simulink model "soal1ghesmatb"  (R2019b)
settings: Solver=VariableStepAuto  StartTime=0.0  StopTime=10.0  RelTol=1e-3
libraries: simulink x2
settings Model: Creator=user  LastModifiedBy=user

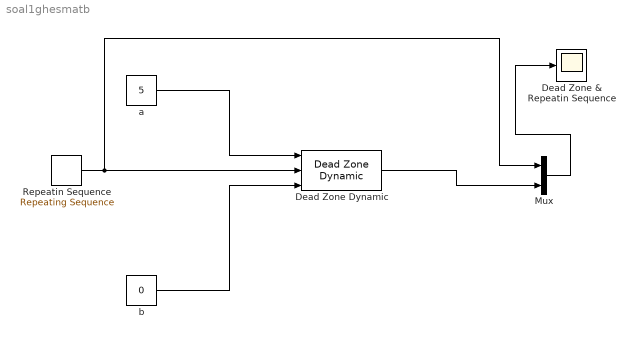
== system soal1ghesmatb ==
  Dead Zone Dynamic : simulink/Discontinuities/Dead Zone Dynamic
      settings: SourceProductName=Simulink  SourceProductBaseCode=SL
  "Dead Zone & Repeatin Sequence " : Scope
  Mux : Mux  Inputs=2
  Repeatin Sequence : simulink/Sources/Repeating Sequence  rep_seq_t=[0 5]  rep_seq_y=[-10 10]
  a : Constant  Value=5
  b : Constant  Value=0
  wires:
  Repeatin Sequence/1 -> Dead Zone Dynamic/2, Mux/1
  b/1 -> Dead Zone Dynamic/3
  a/1 -> Dead Zone Dynamic/1
  Dead Zone Dynamic/1 -> Mux/2
  Mux/1 -> "Dead Zone & Repeatin Sequence "/1
